simulink model "photorealisticSimulationEngi"  (R2025b)
settings: Solver=FixedStepAuto  StartTime=0.0  StopTime=50  RelTol=1e-3  EnableMultiTasking=on
undefined symbols (not defined in the file): Sim3dSensor, UAVSampleTime
libraries: robotcorelib x1, uavutilslib x1, sim3dcameralib x1, sim3dphyssensorlib x1, sim3dlib x1, uavsim3dlib x1
settings Model: DataDictionary=uavPackageDeliveryDataDict.sldd  ModifiedByFormat=The MathWorks, Inc.  Creator=The MathWorks, Inc.  LastModifiedBy=The MathWorks, Inc.
settings SolverCC: AlgebraicLoopSolver=TrustRegion  AutoInsertRateTranBlk=on  MaxZcPerStep=1.0
settings DataIOCC: LimitDataPoints=on  SaveOutput=off  SaveTime=off  ReturnWorkspaceOutputs=off
settings OptimizationCC: EnhancedBackFolding=on  PassReuseOutputArgsThreshold=0.0  ZeroExternalMemoryAtStartup=off  ZeroInternalMemoryAtStartup=off  MaxStackSize=64  OptimizeBlockOrder=speed  DifferentSizesBufferReuse=on  OptimizationCustomize=off
settings DebuggingCC: ParameterPrecisionLossMsg=none  ParameterTunabilityLossMsg=error  UnconnectedInputMsg=warning  UnconnectedOutputMsg=warning  UnconnectedLineMsg=warning  AllowSymbolicDim=off  SubsystemReferenceDiagnosticForUnitTest=warning  SFUnexpectedBacktrackingDiag=warning  SFNoUnconditionalDefaultTransitionDiag=warning  SFExecutionAtInitializationDiag=none  ArithmeticOperatorsInVariantConditions=warning
settings HardwareCC: ProdBitPerPointer=32.0  ProdBitPerSizeT=32.0  ProdBitPerPtrDiffT=32.0  ProdLargestAtomicFloat=None  ProdIntDivRoundTo=Undefined  ProdEndianess=Unspecified  ProdWordSize=32.0  ProdHWDeviceType=Generic->Unspecified (assume 32-bit Generic)
settings ModelReferenceCC: EnableRefExpFcnMdlSchedulingChecks=on  ModelReferenceNumInstancesAllowed=Single  PropagateSignalLabelsOutOfModel=off
settings SFSimCC: SimUseLocalCustomCode=off  MATLABDynamicMemAlloc=off  CustomCodeUndefinedFunction=UseInterfaceOnly  SimTargetLang=C++  SimDLTargetLibrary=mkl-dnn
settings RTWCC: GenerateReport=on  RTWUseLocalCustomCode=off  LaunchReport=on  TargetLang=C++  GPUComputeCapability=3.5  DLArmComputeVersion=19.05
settings CodeAppCC: ForceParamTrailComments=on  OperatorAnnotations=on
settings GRTTargetCC: TargetLangStandard=C89/C90 (ANSI)  CodeInterfacePackaging=C++ class  SubcomponentCodeInterfacePackaging=C++ class
settings ConfigComp: CovMetricSettings=dw  CovSaveCumulativeToWorkspaceVar=on  CovSaveSingleToWorkspaceVar=on  CovExternalEMLEnable=off

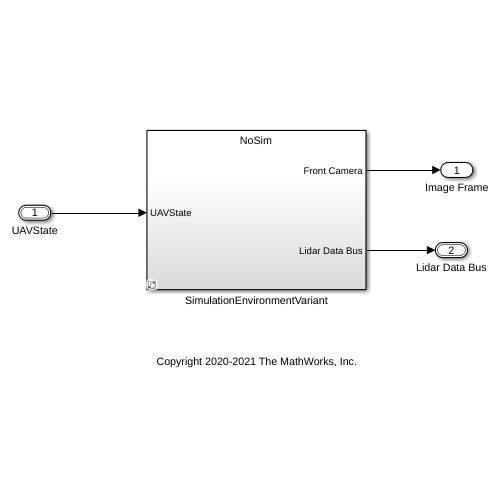
[thumbnail: Simulink's stored preview of the top-level diagram]
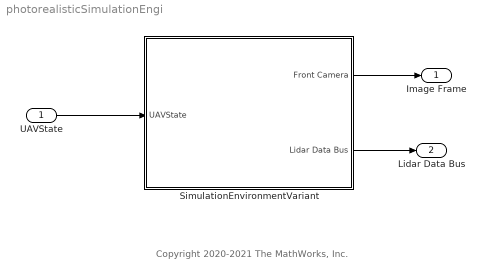
== system photorealisticSimulationEngi ==
  note: Copyright 2020-2021 The MathWorks, Inc.
  UAVState : Inport  OutDataTypeStr=Bus: uavStateBus  BusOutputAsStruct=on
  SimulationEnvironmentVariant : Subsystem  Variant=on  PropagateVariantConditions=on
  Image Frame : Outport
  Lidar Data Bus : Outport  Port=2  OutDataTypeStr=Bus: LidarData
  wires:
  UAVState/1 -> SimulationEnvironmentVariant/1(UAVState)
  SimulationEnvironmentVariant/1(Front Camera) -> Image Frame/1
  SimulationEnvironmentVariant/2(Lidar Data Bus) -> Lidar Data Bus/1

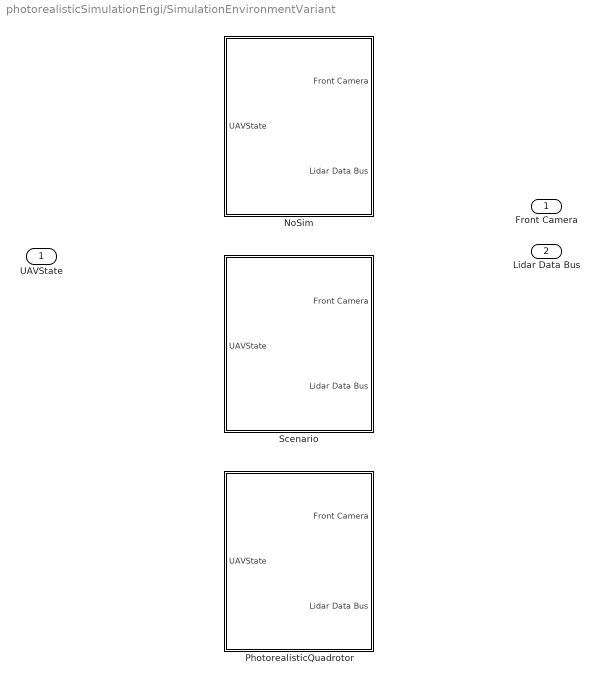
== system photorealisticSimulationEngi/SimulationEnvironmentVariant ==
  UAVState : Inport  OutDataTypeStr=Bus: uavStateBus  PortDimensions=[1 1]  BusOutputAsStruct=on
  NoSim : Subsystem  VariantControl=isPhotoRealisticSim==0
  PhotorealisticQuadrotor : Subsystem  VariantControl=isPhotoRealisticSim==2
  Scenario : Subsystem  VariantControl=isPhotoRealisticSim==1
  Front Camera : Outport  PortDimensions=[ 480 752 3]
  Lidar Data Bus : Outport  Port=2

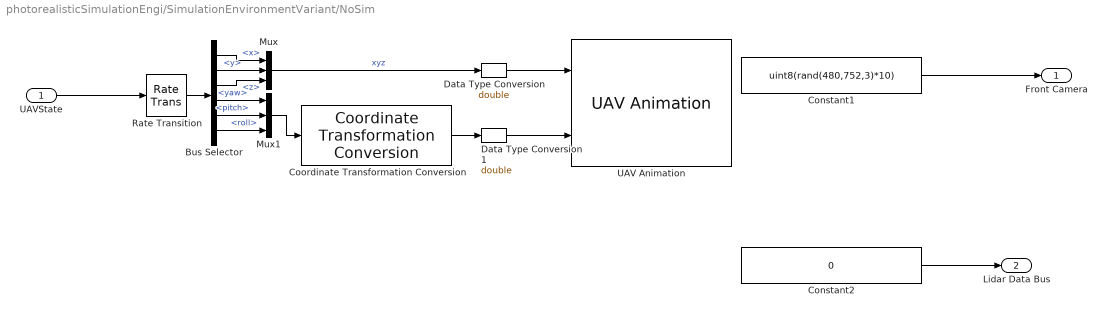
== system photorealisticSimulationEngi/SimulationEnvironmentVariant/NoSim ==
  UAVState : Inport  OutDataTypeStr=Bus: uavStateBus  PortDimensions=[1 1]  SampleTime=UAVSampleTime  BusOutputAsStruct=on
  Bus Selector : BusSelector  OutputSignals=pos_vel.x,pos_vel.y,pos_vel.z,attitude.yaw,attitude.pitch,attitude.roll
  Constant1 : Constant  Value=uint8(rand(480,752,3)*10)
  Constant2 : Constant  Value=0  OutDataTypeStr=Bus: LidarData
  Coordinate Transformation Conversion : robotcorelib/Coordinate Transformation Conversion  InputRepresentation=Euler Angles  InputEulerSequence=ZYX  ShowTrVecInputPort=on  OutputRepresentation=Quaternion  OutputEulerSequence=ZYX  ShowTrVecOutputPort=on  SimulateUsing=Code generation
  Data Type Conversion : DataTypeConversion  OutDataTypeStr=double  SaturateOnIntegerOverflow=off  RndMeth=Floor
  Data Type Conversion1 : DataTypeConversion  OutDataTypeStr=double  SaturateOnIntegerOverflow=off  RndMeth=Floor
  Mux : Mux  Inputs=3
  Mux1 : Mux  Inputs=3
  Rate Transition : RateTransition  OutPortSampleTime=UAVSampleTime*200
  UAV Animation : uavutilslib/UAV Animation  NumUAV=1  DynamicUAVConfig=off  UAVType=Multirotor  UAVSize=1  UAVColor=[1 0 0]  UAVTrajectoryAlpha=1  InertialZDirection=Down  RotationFormat=Quaternion  DrawMarkers=off  SampleTime=UAVSampleTime*200
  Front Camera : Outport  OutDataTypeStr=uint8  PortDimensions=[480 752 3]
  Lidar Data Bus : Outport  Port=2
  wires:
  Constant1/1 -> Front Camera/1
  Constant2/1 -> Lidar Data Bus/1
  Bus Selector/1 -> Mux/1  "<x>"
  Bus Selector/2 -> Mux/2  "<y>"
  Bus Selector/3 -> Mux/3  "<z>"
  Mux/1 -> Data Type Conversion/1  "xyz"
  Bus Selector/6 -> Mux1/3  "<roll>"
  Bus Selector/5 -> Mux1/2  "<pitch>"
  Bus Selector/4 -> Mux1/1  "<yaw>"
  Coordinate Transformation Conversion/1 -> Data Type Conversion1/1
  Mux1/1 -> Coordinate Transformation Conversion/1
  Data Type Conversion1/1 -> UAV Animation/2
  UAVState/1 -> Rate Transition/1
  Data Type Conversion/1 -> UAV Animation/1
  Rate Transition/1 -> Bus Selector/1

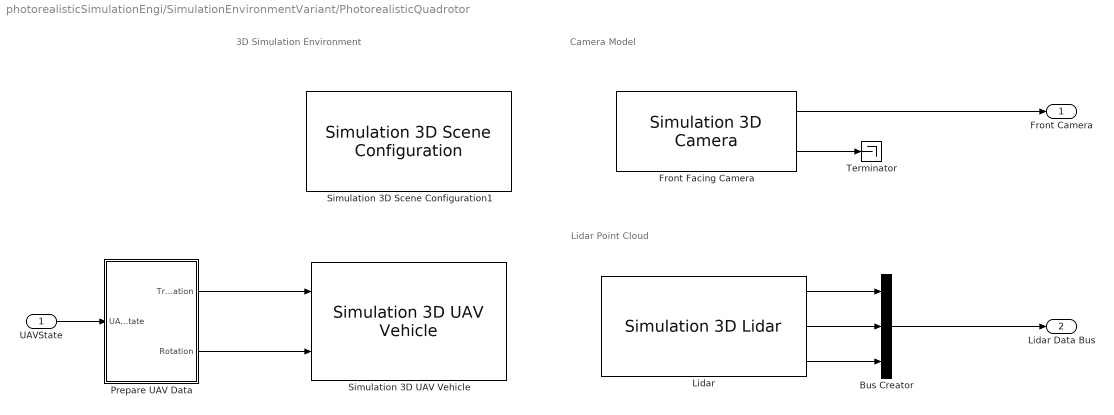
== system photorealisticSimulationEngi/SimulationEnvironmentVariant/PhotorealisticQuadrotor ==
  note: 3D Simulation Environment
  note: Camera Model
  note: Lidar Point Cloud
  UAVState : Inport  PortDimensions=[1 1]  SampleTime=[0.01,0]  BusOutputAsStruct=on
  Bus Creator : BusCreator  Inputs=3  OutDataTypeStr=Bus: LidarData  NonVirtualBus=on
      settings: InheritFromInputs=off
  Front Facing Camera : sim3dcameralib/Simulation 3D Camera  Priority=1  sensorTag=Sim3dSensor�  sensorId=2  sensorName=Sim3dSensor�  vehTagList={'Scene Origin';'SimulinkVehicle1'}  vehTag=SimulinkVehicle1  CoordinateSystem=ISO8855  mountLoc=Origin  offsetFlag=on  tmountOffset=[0 0 -0.15]  extTmount=off  rmountOffset=[0, 0, 0]  extRmount=off  FocalLength=[1109, 1109]  OpticalCenter=[376, 240]  ImageSize=[480, 752]  RadialDistortion=[0, 0]  TangentialDistortion=[0, 0]  SensorSkew=0  VisualizeFieldOfView=off  FieldOfViewRange=61  DepthOutportEnabled=on  SemanticOutportEnabled=off  TransformOutportEnabled=off  SampleTime=UAVSampleTime*20  mountPoint=[0 0 -0.15]  mountOrientation=[0 0 0]  aMode=4  ID=2
      settings: LibrarySourceBlock=uavsim3dlib/Simulation 3D Camera
  Lidar : sim3dphyssensorlib/Simulation 3D Lidar  Priority=1  sensorTag=Sim3dSensor�  sensorId=3  sensorName=Sim3dSensor�  vehTagList={'Scene Origin';'SimulinkVehicle1'}  vehTag=SimulinkVehicle1  CoordinateSystem=ISO8855  mountLoc=Origin  offsetFlag=on  tmountOffset=[0, 0, 0.35]  rmountOffset=[0, 0, 0]  DetectionRange=90  RangeResolution=0.002  VerticalFOV=40  VerticalResolution=1.25  HorizontalFOV=360  HorizontalResolution=0.332409972299169  DistanceOutportEnabled=off  ReflectivityOutportEnabled=off  SemanticOutportEnabled=off  TransformOutportEnabled=on  SampleTime=UAVSampleTime*100  mountPoint=[0 0 0.35]  mountOrientation=[0 0 0]  aMode=4  ID=3
      settings: LibrarySourceBlock=uavsim3dlib/Simulation 3D Lidar
  Prepare UAV Data : Subsystem
  Simulation 3D Scene Configuration1 : sim3dlib/Simulation 3D Scene Configuration  Priority=0  ProjectFormat=Default Scenes  SceneDesc=US city block  ProjectName=/mathworks/devel/bat/filer/batfs2566-0/Bdoc25b.3168145/build/runnable/matlab/toolbox/shared/sim3d_projects/automotive_project_linux/UE/LinuxNoEditor/VehicleSimulation.sh  ScenePath=/Game/Maps/HwStrght  EnableOpenDRIVE=off  vehTagList={'Scene Origin';'SimulinkVehicle1'}  vehTag=SimulinkVehicle1  AttachedCameraRelativeTranslation=[0 0 0]  FreeCameraDefaultInitialTranslation=[-6, 0, 2]  AttachedCameraRelativeRotation=[0 0 0]  FreeCameraDefaultInitialRotation=[0, -15, 0]  ViewpointName=Custom  FreeCameraInitialTranslation=[0 0 0]  ViewpointTranslation=[0 0 0]  FreeCameraInitialRotation=[0 0 0]  ViewpointRotation=[0 0 0]  OpVisEn=off  Ts=0.1  EnableWindow=on  EnableRemoteAccess=off  EnableWeather=off  SunAzimuth=90  SunAltitude=40.0  EnableGeospatialSun=off  Latitude=0  Longitude=0  Date=2023-01-01  Time=10:30:00  GeoTimeZone=-5.0  SunDaylightSaving=off  wind=1  clouds=10  EnableVolumetricClouds=off  CloudCoverage=0  CloudAltitude=6  fog=0  rain=0  RaindropsEffect=off  SnowDensity=0  EnableGeospatial=off  TilesetSource=Earth terrain  UseTrueOrigin=off  OriginHeight=200  OriginLatitude=40.744652  OriginLongitude=-73.988864  MapStyle=Aerial  AdditionalAssetIDs=[]  UseAdvancedSunSky=off  SolarTime=11  TimeZone=-5  Day=21  Month=9  Year=2022  UseDaylightSavingTime=on  DSTStartDay=10  DSTStartMonth=3  DSTEndDay=3  DSTEndMonth=11  DSTSwitchHour=2  sensorTag=MainCamera5  sensorId=5  sensorName=MainCamera5  mountLoc=Origin  offsetFlag=off  tmountOffset=[0, 0, 0]  rmountOffset=[0, 0, 0]  HorizontalResolution=1280  VerticalResolution=720  HorizontalFOV=60  mountPoint=[0 0 0]  mountOrientation=[0 0 0]  aMode=4  ID=5  GeoTrigger=Inactive  ViewNameList={'Custom'}  ViewTranslationList={'[0 0 0]'}  ViewRotationList={'[0 0 0]'}
      settings: LibrarySourceBlock=uavsim3dlib/Simulation 3D Scene Configuration
  Simulation 3D UAV Vehicle : uavsim3dlib/Simulation 3D UAV Vehicle  Mesh=Quadrotor  MeshPath=/MathWorksUAVContent/UAVs/HexaRotorUAV/HexaRotor.HexaRotor  Color=Blue  ActorName=SimulinkVehicle1  UseGlobalFrame=off  InitialTranslation=[-186 105 0]  InitialRotation=[0 0 0]  InitialTranslationGlobal=[0 0 0]  InitialGeoOrigin=[0 0 0]  InitialRotationGlobal=[0 0 0]  SampleTime=-1  ActorType=SimulinkVehicle  ID=1  aMode=4  ActorTag=SimulinkVehicle1
  Terminator : Terminator
  Front Camera : Outport  PortDimensions=[ 480 752 3]
  Lidar Data Bus : Outport  Port=2
  wires:
  Front Facing Camera/1 -> Front Camera/1
  Lidar/1 -> Bus Creator/1
  Lidar/2 -> Bus Creator/2
  Lidar/3 -> Bus Creator/3
  Bus Creator/1 -> Lidar Data Bus/1
  UAVState/1 -> Prepare UAV Data/1(UAVState)
  Front Facing Camera/2 -> Terminator/1
  Prepare UAV Data/1(Translation) -> Simulation 3D UAV Vehicle/1
  Prepare UAV Data/2(Rotation) -> Simulation 3D UAV Vehicle/2

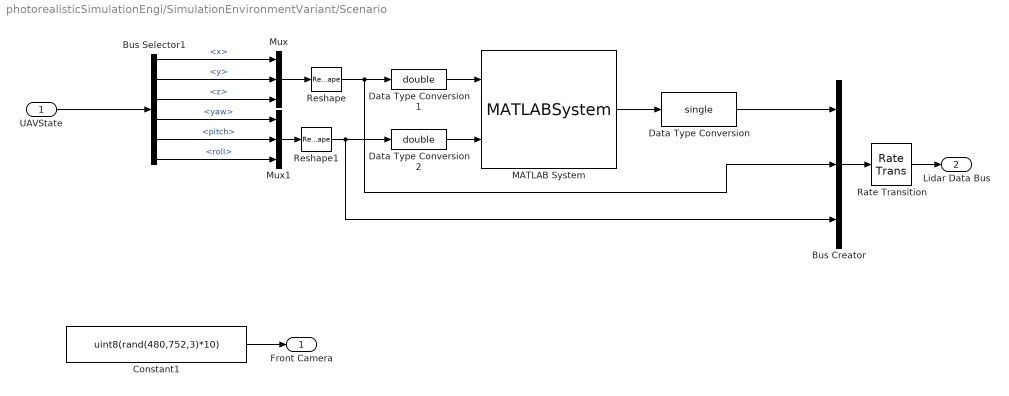
== system photorealisticSimulationEngi/SimulationEnvironmentVariant/Scenario ==
  UAVState : Inport
  Bus Creator : BusCreator  Inputs=3  OutDataTypeStr=Bus: LidarData  NonVirtualBus=on
      settings: InheritFromInputs=off
  Bus Selector1 : BusSelector  OutputSignals=pos_vel.x,pos_vel.y,pos_vel.z,attitude.yaw,attitude.pitch,attitude.roll
  Constant1 : Constant  Value=uint8(rand(480,752,3)*10)
  Data Type Conversion : DataTypeConversion  OutDataTypeStr=single  SaturateOnIntegerOverflow=off  RndMeth=Floor
  Data Type Conversion1 : DataTypeConversion  OutDataTypeStr=double  SaturateOnIntegerOverflow=off  RndMeth=Floor
  Data Type Conversion2 : DataTypeConversion  OutDataTypeStr=double  SaturateOnIntegerOverflow=off  RndMeth=Floor
  MATLAB System : MATLABSystem  System=uavScenarioBlock  InitialPosition=initialConditions.posNED  InitialOrientation=[0 0 0]
      mask Type: uavScenarioBlock
  Mux : Mux  Inputs=3
  Mux1 : Mux  Inputs=3
  Rate Transition : RateTransition  OutPortSampleTime=0.5
  Reshape : Reshape  OutputDimensionality=Row vector (2-D)
  Reshape1 : Reshape  OutputDimensionality=Row vector (2-D)
  Front Camera : Outport
  Lidar Data Bus : Outport  Port=2
  wires:
  Bus Selector1/4 -> Mux1/1  "<yaw>"
  Bus Selector1/2 -> Mux/2  "<y>"
  Bus Selector1/6 -> Mux1/3  "<roll>"
  Bus Selector1/3 -> Mux/3  "<z>"
  Bus Selector1/1 -> Mux/1  "<x>"
  UAVState/1 -> Bus Selector1/1
  Bus Selector1/5 -> Mux1/2  "<pitch>"
  Constant1/1 -> Front Camera/1
  Bus Creator/1 -> Rate Transition/1
  MATLAB System/1 -> Data Type Conversion/1
  Mux/1 -> Reshape/1
  Mux1/1 -> Reshape1/1
  Data Type Conversion1/1 -> MATLAB System/1
  Data Type Conversion2/1 -> MATLAB System/2
  Reshape/1 -> Bus Creator/2, Data Type Conversion1/1
  Reshape1/1 -> Bus Creator/3, Data Type Conversion2/1
  Data Type Conversion/1 -> Bus Creator/1
  Rate Transition/1 -> Lidar Data Bus/1

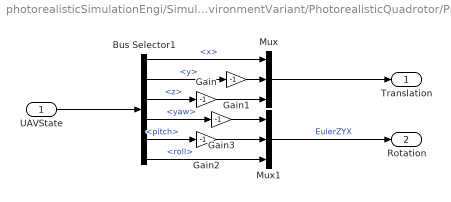
== system photorealisticSimulationEngi/SimulationEnvironmentVariant/PhotorealisticQuadrotor/Prepare UAV Data ==
  UAVState : Inport
  Bus Selector1 : BusSelector  OutputSignals=pos_vel.x,pos_vel.y,pos_vel.z,attitude.yaw,attitude.pitch,attitude.roll
  Gain{,1..3} (4 alike) : Gain  Gain=-1
  Mux : Mux  Inputs=3
  Mux1 : Mux  Inputs=3
  Translation : Outport
  Rotation : Outport  Port=2
  wires:
  UAVState/1 -> Bus Selector1/1
  Mux/1 -> Translation/1
  Mux1/1 -> Rotation/1  "EulerZYX"
  Bus Selector1/4 -> Gain3/1  "<yaw>"
  Bus Selector1/5 -> Gain2/1  "<pitch>"
  Bus Selector1/6 -> Mux1/3  "<roll>"
  Bus Selector1/3 -> Gain/1  "<z>"
  Bus Selector1/2 -> Gain1/1  "<y>"
  Bus Selector1/1 -> Mux/1  "<x>"
  Gain/1 -> Mux/3
  Gain1/1 -> Mux/2
  Gain2/1 -> Mux1/2
  Gain3/1 -> Mux1/1
